simulink model "Controllo_assex_4gdl_discretizzato"  (R2021a)
settings: Solver=VariableStepAuto  StartTime=0.0  StopTime=1.5  RelTol=1e-3
values from neighbouring files (symbols this model uses):
  m = config_dc(parx)    [main.m]
  parx = parametri()    [main.m]
undefined symbols (not defined in the file or in its folder): accelerazioni, Evaluate_Trajectory
libraries: cstblocks x10, simulink x2
settings Model: Creator=user  LastModifiedBy=stefa
settings SolverCC: AlgebraicLoopSolver=TrustRegion
settings DebuggingCC: SFMachineParentedDataDiag=warning

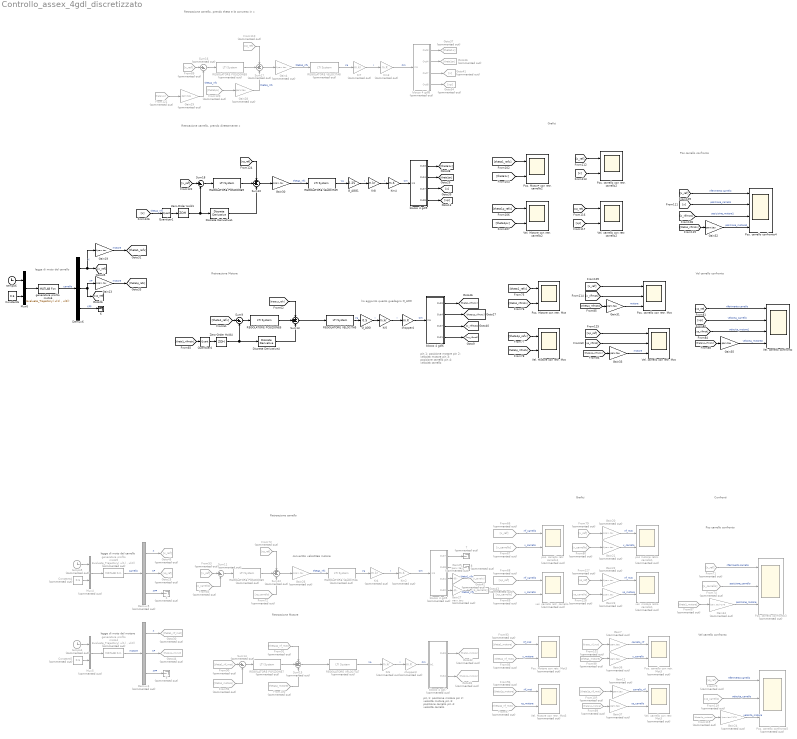
== system Controllo_assex_4gdl_discretizzato ==
  note: ho aggiunto questo guadagno G_AGG
  note: Retroazione carrello, prendo theta e la converto in x
  note: Pos carrello confronto
  note: Retroazione Motore
  note: convertito velcotitaà motore
  note: Vel carrello confronto
  note: Grafici
  note: pin 1: posizione motore
      | pin 2: velocità motore
      | pin 3: posizione carrello
      | pin 4: velocità carrello
  note: legge di moto del carrello
  note: legge di moto del carrello
  note: legge di moto del motore
  note: Grafici
  note: Retroazione carrello
  note: Confronti
  note: Vel carrello confronto
  note: Pos carrello confronto
  note: Retroazione carrello, prendo direttamente x
  note: Retroazione Motore
  note: pin 1: posizione motore
      | pin 2: velocità motore
      | pin 3: posizione carrello
      | pin 4: velocità carrello
   {4..5,7..8} (4 alike) : Terminator  Commented=on
  " 6" : Terminator
  Constant4 : Constant  Commented=on  Value=0.6
  Constant5 : Constant  Commented=on  Value=0.6
  Constant6 : Constant  Value=0.6
  Demux4 : Demux  Commented=on  Outputs=3
  Demux5 : Demux  Commented=on  Outputs=3
  Demux6 : Demux  Outputs=3
  Discrete Derivative1 : simulink/Discrete/Discrete Derivative  gainval=1  ICPrevScaledInput=0.0  OutMin=[]  OutMax=[]  OutDataType=fixdt(1, 16)  OutScaling=2^-10  DoSatur=off
  Discrete Derivative4 : simulink/Discrete/Discrete Derivative  gainval=1.0  ICPrevScaledInput=0.0  OutMin=[]  OutMax=[]  OutDataType=fixdt(1, 16)  OutScaling=2^-10  DoSatur=off
  From{96,99..100,119} (4 alike) : From  Commented=on  GotoTag=theta1p_motore
  From101 : From  Commented=on  GotoTag=theta1_rif_mot
  From103 : From  Commented=on  GotoTag=theta1p_rif_mot
  From{68,70,73,110,127} (5 alike) : From  Commented=on  GotoTag=xp_ref
  From{69,72,118,128} (4 alike) : From  Commented=on  GotoTag=xp_carrello
  From120 : From  Commented=on  GotoTag=theta1px
  From121 : From  Commented=on  GotoTag=theta1px
  From{53,66,71,79,89} (5 alike) : From  Commented=on  GotoTag=x_ref
  From{67,74,80,83} (4 alike) : From  Commented=on  GotoTag=x_carrello
  From{87,92..93,98} (4 alike) : From  Commented=on  GotoTag=theta1_motore
  From90 : From  Commented=on  GotoTag=theta1_rif_mot
  From91 : From  Commented=on  GotoTag=theta1p_rif_mot
  From95 : From  Commented=on  GotoTag=theta1_rif_mot
  From97 : From  Commented=on  GotoTag=theta1p_rif_mot
  G_AGG : Gain  Gain=0.5
  G_AGG1 : Gain  Gain=0.25
  Gain{7,12,25,27..29,36..37} (8 alike) : Gain  Commented=on  Gain=parx.tau
  Gain13 : Gain  Gain=1/parx.tau
  Gain19 : Gain  Gain=1/parx.tau
  Gain{4,20..23,26} (6 alike) : Gain  Commented=on  Gain=1/parx.tau
  Gain24 : Gain  Commented=on  Gain=(parx.tau)*178
  Gain30 : Gain  Gain=1/parx.tau
  Gain{31..33,35} (4 alike) : Gain  Gain=parx.tau
  Gain34 : Gain  Commented=on  Gain=(parx.tau)*178
  Goto25 : Goto  Commented=on  GotoTag=xp_ref
  Goto28 : Goto  Commented=on  GotoTag=theta1p_motore
  Goto30 : Goto  Commented=on  GotoTag=theta1_rif_mot
  Goto32 : Goto  Commented=on  GotoTag=theta1_motore
  Goto34 : Goto  Commented=on  GotoTag=xp
  Goto36 : Goto  Commented=on  GotoTag=theta1px
  Goto37 : Goto  Commented=on  GotoTag=theta1x
  Goto41 : Goto  Commented=on  GotoTag=x
  Goto42 : Goto  Commented=on  GotoTag=x_carrello
  Goto43 : Goto  Commented=on  GotoTag=xp_carrello
  Goto44 : Goto  Commented=on  GotoTag=theta1p_rif_mot
  Goto45 : Goto  Commented=on  GotoTag=x_ref
  Km2 : Gain  Commented=on  Gain=m.K
  Km3 : Gain  Commented=on  Gain=m.K
  Km4 : Gain  Gain=m.K
  Kr4 : Gain  Commented=on  Gain=m.kr
  Kr5 : Gain  Gain=m.kr
  Kr6 : Gain  Commented=on  Gain=m.kr
  Kr7 : Gain  Commented=on  Gain=m.kr
  Kr8 : Gain  Gain=m.kr
  Mux4 : Mux  Commented=on  Inputs=2
  Mux5 : Mux  Commented=on  Inputs=2
  Mux6 : Mux  Inputs=2
  Pos. Motore con retr. Mot : Scope  NumInputPorts=2
  Pos. Motore con retr. Mot3 : Scope  Commented=on  NumInputPorts=2
  Pos. Motore con retr. carrello2 : Scope  NumInputPorts=2
  Pos. carrello con retr. Mot : Scope  NumInputPorts=3
  Pos. carrello con retr. Mot3 : Scope  Commented=on  NumInputPorts=2
  Pos. carrello con retr. carrello2 : Scope  NumInputPorts=2
  Pos. carrello confronto3 : Scope  Commented=on  NumInputPorts=3
  Pos. carrello confronto4 : Scope  NumInputPorts=4
  Pos. carrello confronto5 : Scope  Commented=on  NumInputPorts=3
  Quantizer1 : Quantizer  QuantizationInterval=10/4096
  Quantizer4 : Quantizer  QuantizationInterval=10/4096
  REGOLATORE POSIZIONE5 : cstblocks/LTI System  Commented=on  sys=ap.H_P  IC=[]
  REGOLATORE POSIZIONE6 : cstblocks/LTI System  sys=ap.H_P  IC=[]
  REGOLATORE POSIZIONE7 : cstblocks/LTI System  Commented=on  sys=ap.H_P  IC=[]
  REGOLATORE POSIZIONE8 : cstblocks/LTI System  Commented=on  sys=ap.H_P  IC=[]
  REGOLATORE POSIZIONE9 : cstblocks/LTI System  sys=ap.H_P  IC=[]
  REGOLATORE VELOCITA5 : cstblocks/LTI System  sys=av.PI_V  IC=[]
  REGOLATORE VELOCITA6 : cstblocks/LTI System  Commented=on  sys=av.PI_V  IC=[]
  REGOLATORE VELOCITA7 : cstblocks/LTI System  Commented=on  sys=av.PI_V  IC=[]
  REGOLATORE VELOCITA8 : cstblocks/LTI System  Commented=on  sys=av.PI_V  IC=[]
  REGOLATORE VELOCITA9 : cstblocks/LTI System  sys=av.PI_V  IC=[]
  Sum10 : Sum  Inputs=++-
  Sum11 : Sum  Commented=on  Inputs=|+-
  Sum12 : Sum  Commented=on  Inputs=++-
  Sum13 : Sum  Inputs=++-
  Sum14 : Sum  Commented=on  Inputs=|+-
  Sum15 : Sum  Commented=on  Inputs=++-
  Sum16 : Sum  Commented=on  Inputs=|+-
  Sum17 : Sum  Commented=on  Inputs=++-
  Sum18 : Sum  Inputs=|+-
  Sum9 : Sum  Inputs=|+-
  Vel. Motore con retr. Mot : Scope  NumInputPorts=2
  Vel. Motore con retr. Mot3 : Scope  Commented=on  NumInputPorts=2
  Vel. Motore con retr. carrello2 : Scope  NumInputPorts=2
  Vel. carrello con retr. Mot : Scope  NumInputPorts=3
  Vel. carrello con retr. Mot3 : Scope  Commented=on  NumInputPorts=2
  Vel. carrello con retr. carrello2 : Scope  NumInputPorts=2
  Vel. carrello confronto : Scope  NumInputPorts=4
  Zero-Order Hold1 : ZeroOrderHold  SampleTime=0.001
  Zero-Order Hold4 : ZeroOrderHold  SampleTime=0.001
  blocco 4 gdl5 : Subsystem  Commented=on
  blocco 4 gdl6 : Subsystem
  blocco 4 gdl7 : Subsystem  Commented=on
  blocco 4 gdl8 : Subsystem  Commented=on
  blocco 4 gdl9 : Subsystem
  chopper3 : Gain  Commented=on  Gain=m.K
  chopper4 : Gain  Gain=m.K
  generatore profilo moto4 : MATLABFcn  Commented=on  MATLABFcn=Evaluate_Trajectory( u(1) , u(2))  OutputDimensions=3
  generatore profilo moto5 : MATLABFcn  Commented=on  MATLABFcn=Evaluate_Trajectory( u(1) , u(2))  OutputDimensions=3
  generatore profilo moto6 : MATLABFcn  MATLABFcn=Evaluate_Trajectory( u(1) , u(2))  OutputDimensions=3
  pos motore retro. carrello1 : Scope  Commented=on  NumInputPorts=2
  pos. carrello retr. carrello1 : Scope  Commented=on  NumInputPorts=2
  tempo4 : Clock  Commented=on
  tempo5 : Clock  Commented=on
  tempo6 : Clock
  vel. carrello retr. carrello1 : Scope  Commented=on  NumInputPorts=2
  vel. motore retro. carrello1 : Scope  Commented=on  NumInputPorts=2
  wires:
  Kr4/1 -> Km2/1  "I"
  blocco 4 gdl9/1(Out3) -> [theta1x]
  Gain24/1 -> Pos. carrello confronto5/3  "velocita_motore"
  [theta1_refx] -> Pos. Motore con retr. carrello2/1
  blocco 4 gdl9/2(Out4) -> [theta1px]
  From103/1 -> Gain12/1
  blocco 4 gdl8/3(Out7) -> Goto41/1
  Kr8/1 -> Km4/1  "I"
  [theta1_refx] -> Pos. Motore con retr. Mot/1
  [theta1_refx] -> Sum9/1
  Constant4/1 -> Mux4/2
  [xp] -> Vel. carrello confronto/2  "velocita_carrello"
  blocco 4 gdl9/3(Out7) -> [x]
  From119/1 -> Gain24/1
  Sum14/1 -> REGOLATORE POSIZIONE7/1
  Gain20/1 -> pos motore retro. carrello1/1  "rif_mot"
  Gain27/1 -> Goto43/1  "theta1_rifx"
  From118/1 -> Pos. carrello confronto5/2  "velocita_carrello"
  From120/1 -> Gain28/1
  Sum18/1 -> REGOLATORE POSIZIONE9/1
  [xp_ref] -> Sum10/1
  Gain29/1 -> Sum16/2  "theta1_rifx"
  Gain22/1 -> vel. motore retro. carrello1/1  "rif_mot"
  From71/1 -> Pos. carrello confronto3/1  "riferimento carrello"
  [x_ref] -> Sum18/1
  Gain31/1 -> Pos. carrello con retr. Mot/3  "motore"
  From87/1 -> Gain34/1
  From127/1 -> Gain22/1
  Gain36/1 -> Pos. carrello con retr. Mot3/2  "x_carrello"
  Constant5/1 -> Mux5/2
  Km4/1 -> blocco 4 gdl9/1(In1)  "Cm"
  blocco 4 gdl9/4(Out8) -> [xp]
  Gain13/1 -> [theta1p_refx]  "motore"
  REGOLATORE VELOCITA8/1 -> Kr7/1  "Va"
  Kr7/1 -> Km3/1  "I"
  REGOLATORE POSIZIONE9/1 -> Sum10/2
  Km3/1 -> blocco 4 gdl8/1(In1)  "Cm"
  [x] -> Pos. carrello confronto4/2  "posizione_carrello"
  From70/1 -> Pos. carrello confronto5/1  "riferimento carrello"
  Sum10/1 -> Gain30/1
  From72/1 -> Sum12/3
  Km2/1 -> blocco 4 gdl5/1(In1)  "Cm"
  From89/1 -> Sum16/1
  Gain23/1 -> vel. motore retro. carrello1/2  "xp_motore"
  [theta1p_rifmotx] -> Gain35/1
  From66/1 -> pos. carrello retr. carrello1/1  "rif_carrello"
  Demux6/3 -> " 6"/1  "XPP"
  From128/1 -> Gain23/1
  [theta1_rifmotx] -> Pos. Motore con retr. Mot/2
  From121/1 -> Gain29/1
  [xp] -> Vel. carrello con retr. carrello2/2
  blocco 4 gdl5/4(Out2) -> Gain27/1
  blocco 4 gdl5/2(Out8) -> " 8"/1
  Gain28/1 -> Sum17/3  "theta1_rifx"
  From80/1 -> Gain21/1
  blocco 4 gdl5/3(Out1) -> Gain25/1
  Sum16/1 -> REGOLATORE POSIZIONE8/1
  Gain19/1 -> [theta1_refx]  "motore"
  Gain21/1 -> pos motore retro. carrello1/2  "x_carrello"
  [theta1_rifmotx] -> Gain32/1
  [x] -> Pos. carrello con retr. carrello2/2
  From79/1 -> Gain20/1
  Gain4/1 -> REGOLATORE VELOCITA8/1  "theta1_rifx"
  [x_ref] -> Pos. carrello con retr. carrello2/1
  [theta1p_rifmotx] -> Gain33/1
  [xp_ref] -> Vel. carrello con retr. carrello2/1
  Kr6/1 -> chopper3/1  "I"
  REGOLATORE POSIZIONE8/1 -> Sum17/2
  Sum17/1 -> Gain4/1
  REGOLATORE POSIZIONE7/1 -> Sum15/2
  From93/1 -> Pos. Motore con retr. Mot3/1  "rif_mot"
  [x_ref] -> Pos. carrello confronto4/1  "riferimento carrello"
  From74/1 -> Pos. carrello confronto3/2  "posizione_carrello"
  Mux6/1 -> generatore profilo moto6/1
  From96/1 -> Vel. Motore con retr. Mot3/1  "rif_mot"
  From110/1 -> Sum17/1
  [x_rifmot] -> Pos. carrello confronto4/3  "posizioine_motore1"
  [theta1p_refx] -> Vel. Motore con retr. carrello2/1
  blocco 4 gdl7/2(Out4) -> Goto28/1
  blocco 4 gdl8/1(Out3) -> Goto37/1
  blocco 4 gdl8/2(Out4) -> Goto36/1
  Demux4/1 -> Goto30/1  "X"
  [theta1px] -> Vel. Motore con retr. carrello2/2
  Gain32/1 -> Pos. carrello confronto4/4  "posizione_motore2"
  blocco 4 gdl8/4(Out8) -> Goto34/1
  Constant6/1 -> Mux6/2
  Gain33/1 -> Vel. carrello con retr. Mot/3  "motore"
  Demux4/3 -> " 5"/1  "XPP"
  Gain34/1 -> Pos. carrello confronto3/3  "posizione_motore"
  tempo6/1 -> Mux6/1
  Demux6/2 -> Gain13/1, [xp_ref]  "XP"
  From98/1 -> Gain36/1
  Sum9/1 -> REGOLATORE POSIZIONE6/1
  From97/1 -> Vel. Motore con retr. Mot3/2  "xp_motore"
  chopper4/1 -> blocco 4 gdl6/1(In1)  "Cm"
  blocco 4 gdl6/3(Out7) -> [x_rifmot]
  From92/1 -> Sum14/2
  From90/1 -> Sum14/1
  From100/1 -> Sum15/3
  From101/1 -> Gain7/1
  chopper3/1 -> blocco 4 gdl7/1(In1)  "Cm"
  blocco 4 gdl5/1(Out7) -> " 7"/1
  Gain12/1 -> Vel. carrello con retr. Mot3/1  "carrello_rif"
  From95/1 -> Pos. Motore con retr. Mot3/2  "x_motore"
  blocco 4 gdl7/1(Out3) -> Goto32/1
  Gain37/1 -> Vel. carrello con retr. Mot3/2  "xp_carrello"
  tempo4/1 -> Mux5/1
  [x_rifmot] -> Pos. carrello con retr. Mot/2
  Kr5/1 -> chopper4/1  "I"
  [theta1_rifmotx] -> Gain31/1
  generatore profilo moto4/1 -> Demux4/1  "motore"
  Mux5/1 -> generatore profilo moto4/1
  blocco 4 gdl6/4(Out1) -> [xp_rifmot]
  From67/1 -> pos. carrello retr. carrello1/2  "x_carrello"
  Gain30/1 -> REGOLATORE VELOCITA9/1  "theta1_rifx"
  [xp_rifmot] -> Vel. carrello confronto/3  "velocita_motore1"
  [theta1p_refx] -> Sum13/1
  From91/1 -> Sum15/1
  [xp_ref] -> Vel. carrello confronto/1  "riferimento carrello"
  [x_ref] -> Pos. carrello con retr. Mot/1
  [theta1p_rifmotx] -> Vel. Motore con retr. Mot/2
  [theta1x] -> Pos. Motore con retr. carrello2/2
  Sum13/1 -> REGOLATORE VELOCITA5/1
  [xp_ref] -> Vel. carrello con retr. Mot/1
  From83/1 -> Sum11/2
  From68/1 -> vel. carrello retr. carrello1/1  "rif_carrello"
  From53/1 -> Sum11/1
  From99/1 -> Gain37/1
  REGOLATORE POSIZIONE6/1 -> Sum13/2
  [xp_rifmot] -> Vel. carrello con retr. Mot/2
  blocco 4 gdl6/2(Out4) -> [theta1p_rifmotx]
  blocco 4 gdl6/1(Out3) -> [theta1_rifmotx]
  [theta1p_refx] -> Vel. Motore con retr. Mot/1
  Gain25/1 -> Goto42/1  "theta1_rifx"
  Demux4/2 -> Goto44/1  "XP"
  generatore profilo moto6/1 -> Demux6/1  "carrello"
  Sum12/1 -> Gain26/1
  Gain7/1 -> Pos. carrello con retr. Mot3/1  "carrello_rif"
  Demux5/1 -> Goto45/1  "X"
  Demux5/2 -> Goto25/1  "XP"
  Gain26/1 -> REGOLATORE VELOCITA6/1  "theta1_rifx"
  Sum15/1 -> REGOLATORE VELOCITA7/1
  Sum11/1 -> REGOLATORE POSIZIONE5/1
  Gain35/1 -> Vel. carrello confronto/4  "velocita_motore2"
  REGOLATORE VELOCITA7/1 -> Kr6/1  "Va"
  REGOLATORE POSIZIONE5/1 -> Sum12/2
  From69/1 -> vel. carrello retr. carrello1/2  "x_carrello"
  generatore profilo moto5/1 -> Demux5/1  "carrello"
  Mux4/1 -> generatore profilo moto5/1
  tempo5/1 -> Mux4/1
  Demux5/3 -> " 4"/1  "XPP"
  REGOLATORE VELOCITA6/1 -> Kr4/1  "Va"
  Demux6/1 -> [x_ref], Gain19/1  "X"
  From73/1 -> Sum12/1
  Quantizer1/1 -> Zero-Order Hold1/1
  [x] -> Quantizer1/1  "theta1_rifx"
  Zero-Order Hold1/1 -> Discrete Derivative1/1, Sum18/2
  Discrete Derivative1/1 -> Sum10/3
  Quantizer4/1 -> Zero-Order Hold4/1
  [theta1_rifmotx] -> Quantizer4/1
  Zero-Order Hold4/1 -> Sum9/2, Discrete Derivative4/1
  Discrete Derivative4/1 -> Sum13/3
  REGOLATORE VELOCITA5/1 -> G_AGG/1  "Va"
  G_AGG/1 -> Kr5/1  "I"
  REGOLATORE VELOCITA9/1 -> G_AGG1/1  "Va"
  G_AGG1/1 -> Kr8/1  "I"

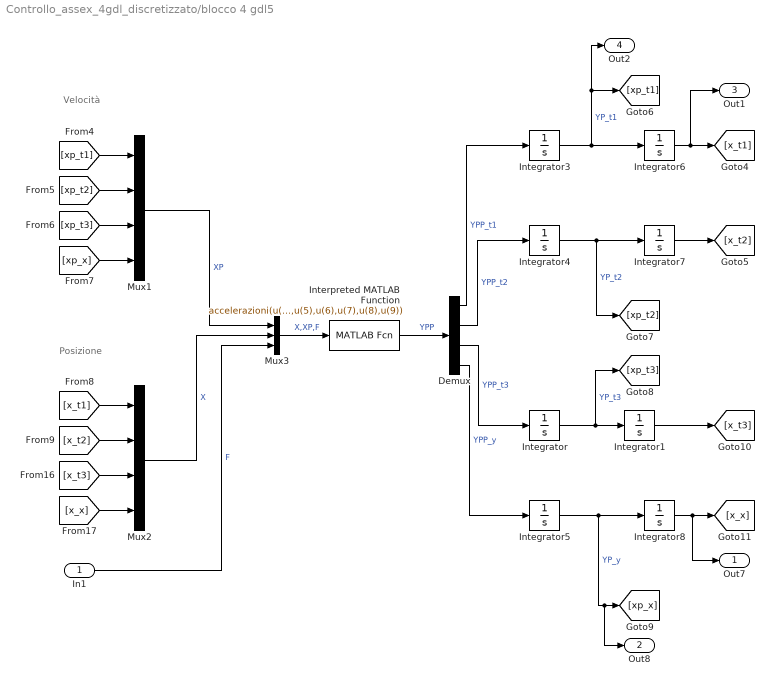
== system Controllo_assex_4gdl_discretizzato/blocco 4 gdl5 ==
  note: Velocità
  note: Posizione
  In1 : Inport
  Demux : Demux
  Integrator{,1,3..8} (8 alike) : Integrator
  Interpreted MATLAB Function : MATLABFcn  MATLABFcn=accelerazioni(u(1),u(2),u(3),u(4),u(5),u(6),u(7),u(8),u(9))  OutputDimensions=4
  Mux1 : Mux
  Mux2 : Mux
  Mux3 : Mux  Inputs=3
  Out7 : Outport
  Out8 : Outport  Port=2
  Out1 : Outport  Port=3
  Out2 : Outport  Port=4
  wires:
  Integrator4/1 -> [xp_t2], Integrator7/1  "YP_t2"
  [xp_t1] -> Mux1/1
  [x_t2] -> Mux2/2
  Integrator1/1 -> [x_t3]
  Demux/4 -> Integrator5/1  "YPP_y"
  Demux/2 -> Integrator4/1  "YPP_t2"
  In1/1 -> Mux3/3  "F"
  Mux3/1 -> Interpreted MATLAB Function/1  "X,XP,F"
  [xp_t2] -> Mux1/2
  Integrator6/1 -> Out1/1, [x_t1]
  Mux2/1 -> Mux3/2  "X"
  Demux/3 -> Integrator/1  "YPP_t3"
  Integrator5/1 -> Out8/1, [xp_x], Integrator8/1  "YP_y"
  Integrator8/1 -> Out7/1, [x_x]
  [xp_x] -> Mux1/4
  [x_x] -> Mux2/4
  Integrator7/1 -> [x_t2]
  Demux/1 -> Integrator3/1  "YPP_t1"
  [x_t1] -> Mux2/1
  Integrator3/1 -> Out2/1, [xp_t1], Integrator6/1  "YP_t1"
  [x_t3] -> Mux2/3
  Interpreted MATLAB Function/1 -> Demux/1  "YPP"
  Mux1/1 -> Mux3/1  "XP"
  Integrator/1 -> Integrator1/1, [xp_t3]  "YP_t3"
  [xp_t3] -> Mux1/3

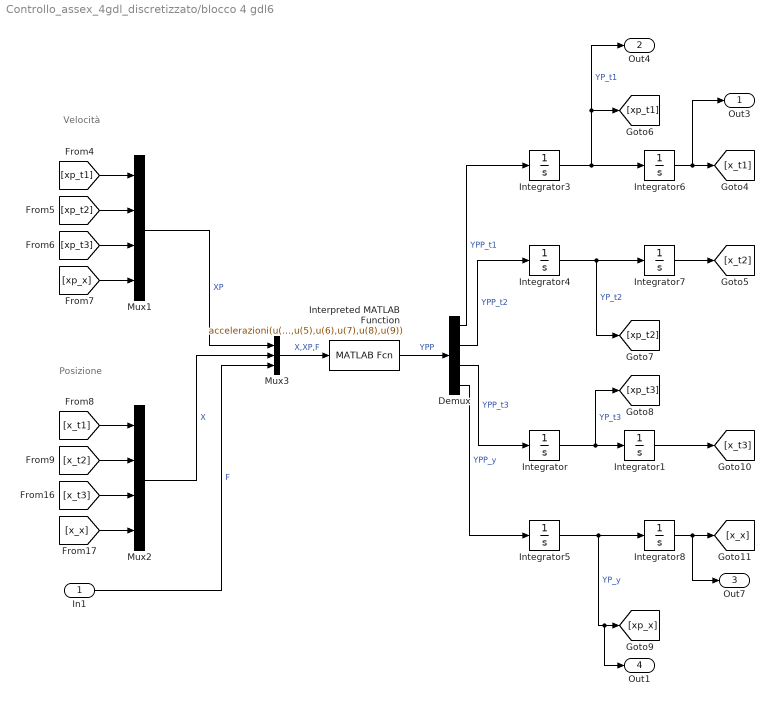
== system Controllo_assex_4gdl_discretizzato/blocco 4 gdl6 ==
  note: Posizione
  note: Velocità
  In1 : Inport
  Demux : Demux
  Integrator{,1,3..7} (7 alike) : Integrator
  Integrator8 : Integrator  InitialCondition=0.0005
  Interpreted MATLAB Function : MATLABFcn  MATLABFcn=accelerazioni(u(1),u(2),u(3),u(4),u(5),u(6),u(7),u(8),u(9))  OutputDimensions=4
  Mux1 : Mux
  Mux2 : Mux
  Mux3 : Mux  Inputs=3
  Out3 : Outport
  Out4 : Outport  Port=2
  Out7 : Outport  Port=3
  Out1 : Outport  Port=4
  wires:
  [xp_t3] -> Mux1/3
  Interpreted MATLAB Function/1 -> Demux/1  "YPP"
  Integrator3/1 -> Out4/1, [xp_t1], Integrator6/1  "YP_t1"
  Integrator8/1 -> Out7/1, [x_x]
  Integrator7/1 -> [x_t2]
  [xp_x] -> Mux1/4
  [x_t1] -> Mux2/1
  Mux1/1 -> Mux3/1  "XP"
  [x_x] -> Mux2/4
  Demux/3 -> Integrator/1  "YPP_t3"
  Integrator/1 -> Integrator1/1, [xp_t3]  "YP_t3"
  Mux2/1 -> Mux3/2  "X"
  Integrator6/1 -> Out3/1, [x_t1]
  Integrator5/1 -> Out1/1, [xp_x], Integrator8/1  "YP_y"
  [xp_t2] -> Mux1/2
  Mux3/1 -> Interpreted MATLAB Function/1  "X,XP,F"
  [x_t3] -> Mux2/3
  In1/1 -> Mux3/3  "F"
  Demux/4 -> Integrator5/1  "YPP_y"
  Integrator4/1 -> [xp_t2], Integrator7/1  "YP_t2"
  Integrator1/1 -> [x_t3]
  [xp_t1] -> Mux1/1
  [x_t2] -> Mux2/2
  Demux/2 -> Integrator4/1  "YPP_t2"
  Demux/1 -> Integrator3/1  "YPP_t1"

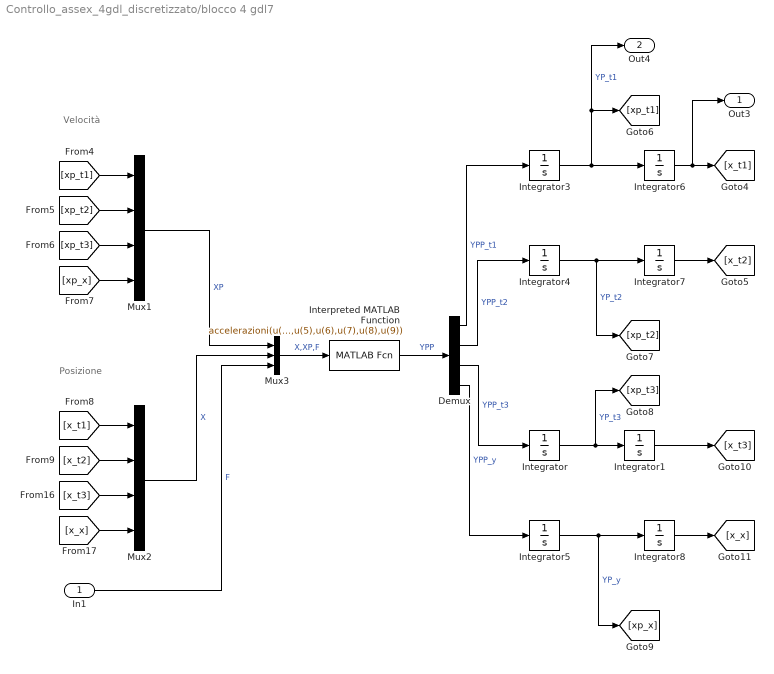
== system Controllo_assex_4gdl_discretizzato/blocco 4 gdl7 ==
  note: Posizione
  note: Velocità
  In1 : Inport
  Demux : Demux
  Integrator{,1,3..8} (8 alike) : Integrator
  Interpreted MATLAB Function : MATLABFcn  MATLABFcn=accelerazioni(u(1),u(2),u(3),u(4),u(5),u(6),u(7),u(8),u(9))  OutputDimensions=4
  Mux1 : Mux
  Mux2 : Mux
  Mux3 : Mux  Inputs=3
  Out3 : Outport
  Out4 : Outport  Port=2
  wires:
  [xp_t3] -> Mux1/3
  Interpreted MATLAB Function/1 -> Demux/1  "YPP"
  Integrator3/1 -> Out4/1, [xp_t1], Integrator6/1  "YP_t1"
  Integrator8/1 -> [x_x]
  Integrator7/1 -> [x_t2]
  [xp_x] -> Mux1/4
  [x_t1] -> Mux2/1
  Mux1/1 -> Mux3/1  "XP"
  [x_x] -> Mux2/4
  Demux/3 -> Integrator/1  "YPP_t3"
  Integrator/1 -> Integrator1/1, [xp_t3]  "YP_t3"
  Mux2/1 -> Mux3/2  "X"
  Integrator6/1 -> Out3/1, [x_t1]
  Integrator5/1 -> [xp_x], Integrator8/1  "YP_y"
  [xp_t2] -> Mux1/2
  Mux3/1 -> Interpreted MATLAB Function/1  "X,XP,F"
  [x_t3] -> Mux2/3
  In1/1 -> Mux3/3  "F"
  Demux/4 -> Integrator5/1  "YPP_y"
  Integrator4/1 -> [xp_t2], Integrator7/1  "YP_t2"
  Integrator1/1 -> [x_t3]
  [xp_t1] -> Mux1/1
  [x_t2] -> Mux2/2
  Demux/2 -> Integrator4/1  "YPP_t2"
  Demux/1 -> Integrator3/1  "YPP_t1"

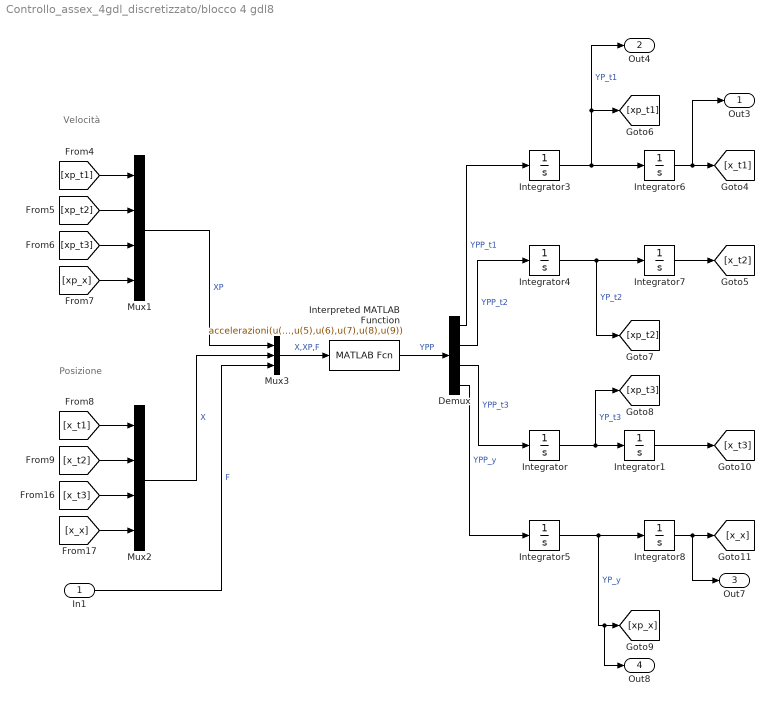
== system Controllo_assex_4gdl_discretizzato/blocco 4 gdl8 ==
  note: Velocità
  note: Posizione
  In1 : Inport
  Demux : Demux
  Integrator{,1,3..7} (7 alike) : Integrator
  Integrator8 : Integrator  InitialCondition=0.0005
  Interpreted MATLAB Function : MATLABFcn  MATLABFcn=accelerazioni(u(1),u(2),u(3),u(4),u(5),u(6),u(7),u(8),u(9))  OutputDimensions=4
  Mux1 : Mux
  Mux2 : Mux
  Mux3 : Mux  Inputs=3
  Out3 : Outport
  Out4 : Outport  Port=2
  Out7 : Outport  Port=3
  Out8 : Outport  Port=4
  wires:
  Integrator4/1 -> [xp_t2], Integrator7/1  "YP_t2"
  [xp_t1] -> Mux1/1
  [x_t2] -> Mux2/2
  Integrator1/1 -> [x_t3]
  Demux/4 -> Integrator5/1  "YPP_y"
  Demux/2 -> Integrator4/1  "YPP_t2"
  In1/1 -> Mux3/3  "F"
  Mux3/1 -> Interpreted MATLAB Function/1  "X,XP,F"
  [xp_t2] -> Mux1/2
  Integrator6/1 -> Out3/1, [x_t1]
  Mux2/1 -> Mux3/2  "X"
  Demux/3 -> Integrator/1  "YPP_t3"
  Integrator5/1 -> Out8/1, [xp_x], Integrator8/1  "YP_y"
  Integrator8/1 -> Out7/1, [x_x]
  [xp_x] -> Mux1/4
  [x_x] -> Mux2/4
  Integrator7/1 -> [x_t2]
  Demux/1 -> Integrator3/1  "YPP_t1"
  [x_t1] -> Mux2/1
  Integrator3/1 -> Out4/1, [xp_t1], Integrator6/1  "YP_t1"
  [x_t3] -> Mux2/3
  Interpreted MATLAB Function/1 -> Demux/1  "YPP"
  Mux1/1 -> Mux3/1  "XP"
  Integrator/1 -> Integrator1/1, [xp_t3]  "YP_t3"
  [xp_t3] -> Mux1/3

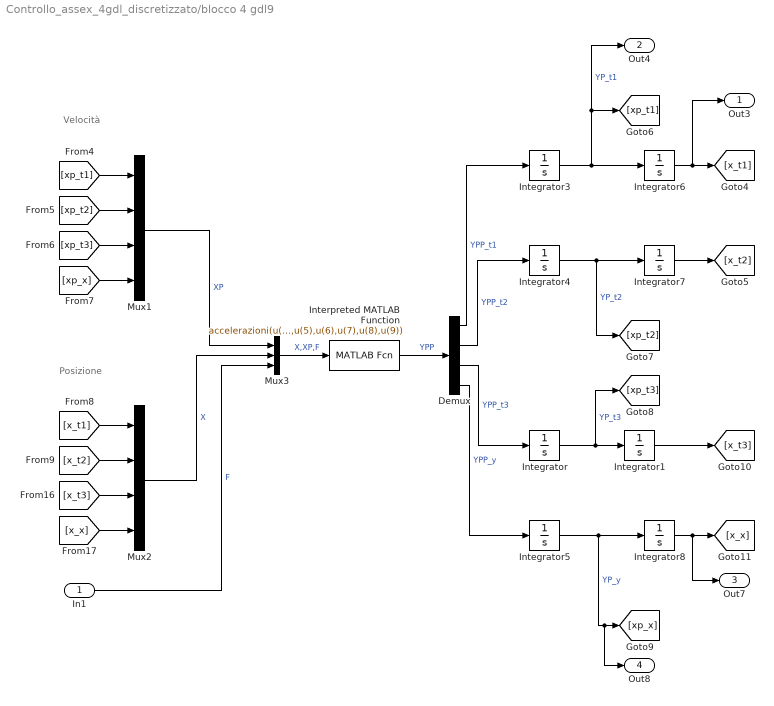
== system Controllo_assex_4gdl_discretizzato/blocco 4 gdl9 ==
  note: Velocità
  note: Posizione
  In1 : Inport
  Demux : Demux
  Integrator{,1,3..7} (7 alike) : Integrator
  Integrator8 : Integrator  InitialCondition=0.0005
  Interpreted MATLAB Function : MATLABFcn  MATLABFcn=accelerazioni(u(1),u(2),u(3),u(4),u(5),u(6),u(7),u(8),u(9))  OutputDimensions=4
  Mux1 : Mux
  Mux2 : Mux
  Mux3 : Mux  Inputs=3
  Out3 : Outport
  Out4 : Outport  Port=2
  Out7 : Outport  Port=3
  Out8 : Outport  Port=4
  wires:
  Integrator4/1 -> [xp_t2], Integrator7/1  "YP_t2"
  [xp_t1] -> Mux1/1
  [x_t2] -> Mux2/2
  Integrator1/1 -> [x_t3]
  Demux/4 -> Integrator5/1  "YPP_y"
  Demux/2 -> Integrator4/1  "YPP_t2"
  In1/1 -> Mux3/3  "F"
  Mux3/1 -> Interpreted MATLAB Function/1  "X,XP,F"
  [xp_t2] -> Mux1/2
  Integrator6/1 -> Out3/1, [x_t1]
  Mux2/1 -> Mux3/2  "X"
  Demux/3 -> Integrator/1  "YPP_t3"
  Integrator5/1 -> Out8/1, [xp_x], Integrator8/1  "YP_y"
  Integrator8/1 -> Out7/1, [x_x]
  [xp_x] -> Mux1/4
  [x_x] -> Mux2/4
  Integrator7/1 -> [x_t2]
  Demux/1 -> Integrator3/1  "YPP_t1"
  [x_t1] -> Mux2/1
  Integrator3/1 -> Out4/1, [xp_t1], Integrator6/1  "YP_t1"
  [x_t3] -> Mux2/3
  Interpreted MATLAB Function/1 -> Demux/1  "YPP"
  Mux1/1 -> Mux3/1  "XP"
  Integrator/1 -> Integrator1/1, [xp_t3]  "YP_t3"
  [xp_t3] -> Mux1/3
